simulink model "CAVE_MachE_speedCtrl"  (R2021b)
settings: configuration reference "ConfigSetDesktopFixedStep" (kept outside this file)
PreLoadFcn:
  | VSS_BICYCLE=Simulink.Variant('Dual=0');
  | VSS_DUAL=Simulink.Variant('Dual=1');
  | Dual=1;
  | load('DriveCycle2.mat')
PostLoadFcn:
  | if any(exist('dsrtsu_mdlpostloadfcn', 'file') ~= 0), dsrtsu_mdlpostloadfcn('Execute', bdroot); end
InitFcn:
  | , if any(exist('rtifpga_mdlclblib', 'file') ~= 0), rtifpga_mdlclblib('Init', bdroot); end,
  | , if any(exist('dsmpb_private', 'file') ~= 0), dsmpb_private('dsmpb_mdlclblib', 'Init', bdroot); end,
  | load('DriveCycle2.mat')
model workspace (MAT data in the model file):
  Gas = 0.383333333333
undefined symbols (not defined in the file or in its folder): AccelCmd, ActTqLF_Nm_, ActTqLR_Nm_, ActTqRF_Nm_, ActTqRR_Nm_, BattChargeLimitMaxPwr, BattChargeLimitSocBpts, BattChargeLimitTbl, BattChrgCapcty, BattDischargeLimitSocBpts, BattDischargeLimitTbl, BattDischargeMaxPwr, BattNumCellsParallel, BattNumCellsSeries, BattOpenVoltCapBpts, BattOpenVoltTbl, BattResistSocBpts, BattResistTbl, BattResistTempBpts, blkCmb_vertType_c1, BrakeMaxPrs, BrakeMaxTrq, ChassisDistCg2FrontAxle, ChassisDistCg2RearAxle, ChassisVehMass, CltchCmd, CoastDown, DecelCmd, DiffRatio, DiscIntNeverNeededParam, EnvGravCnst, EnvPrs, EnvTemp, FuelSpecificGrav, GearCmd, h, InitStates, lgSw, limitedMCT, MCT, MtrEffSpdBpts, MtrEffTbl, MtrEffTrqBpts, MtrPwrMax, MtrTrqMax, pMCT, Ref_speed, Ref_time, SteeringCmd, SupvsryCtrlRegenBrkCutOffTbl, SupvsryCtrlRegenSpdBpts, TestScnrioCycleNum, US06, vdynblks, VEH, vehdyntireFiala
libraries: VSIGenLib x65, simulink x54, etargetslib x38, dsmpblib x24, vehdynlibtire x12, autolibshared x9, vehdynlibsuspension x7, vehdynlibtirecommon x7, autolibutils x5, CarMaker4SL x4, VsrLibWheel x4, autolibpowerinfoutils x3
(part 5 of 14)

== system CAVE_MachE_speedCtrl/Vehicle Under Test/Vehicle/Vehicle Dynamics/Vehicle 14DOF/Brake Pressure ==
  BrkReq : Inport
  Bus Creator1 : BusCreator  Inputs=2
  Gain : Gain  Gain=BrakeMaxPrs
  Gain{1..4} (4 alike) : Gain  Gain=0.5
  Saturation{,1..3} (4 alike) : Saturate  UpperLimit=BrakeMaxPrs  LowerLimit=0  ZeroCross=off
  Signal Specification : SignalSpecification  Unit=Pa
  Terminator : Terminator
  Vector Concatenate2 : Concatenate  NumInputs=4
  BrakePrs : Outport  Unit=Pa
  wires:
  BrkReq/1 -> Gain/1, Bus Creator1/1  "BrkReq"
  Gain/1 -> Signal Specification/1
  Signal Specification/1 -> Gain2/1, Gain1/1, Bus Creator1/2  "BrkPrs"
  Bus Creator1/1 -> Terminator/1  "WhlBrk"
  Gain1/1 -> Gain4/1
  Gain2/1 -> Gain3/1
  Gain3/1 -> Saturation/1, Saturation1/1
  Gain4/1 -> Saturation2/1, Saturation3/1
  Vector Concatenate2/1 -> BrakePrs/1
  Saturation/1 -> Vector Concatenate2/1
  Saturation1/1 -> Vector Concatenate2/2
  Saturation2/1 -> Vector Concatenate2/3
  Saturation3/1 -> Vector Concatenate2/4

== system CAVE_MachE_speedCtrl/Vehicle Under Test/Vehicle/Vehicle Dynamics/Vehicle 14DOF/Steering ==
  SteeringCmd : Inport
  Constant : Constant  Value=0
  Kinematic Steering : vehdynlibsteering/Kinematic Steering  StrgType=Parallel  StrgRatioType=Constant  Loc=Front  NrmlFctr=1  TrckWdth=1.9  WhlBase=ChassisDistCg2FrontAxle+ChassisDistCg2RearAxle  Db=0  StrgRng=2.91*pi  StrgAngBpts="[-6.2832   -5.0265   -3.7699   -2.5133   -1.2566         0    1.2566    2.5133    3.7699    5.0265    6.2832]"  StrgRatioTbl=|  StrgRatio=16.8  StrgArmLngth=0.1  RckCsLngth=0.5  TieRodLngth=0.248  D=0.2  PnnRadius=0.0057  PnnRadiusTbl="[0.0055    0.0055    0.0056    0.0057    0.0058    0.0057    0.0057    0.0057    0.0056    0.0055    0.0055]"  RodLngth=0.1  ParaArmLngth=0.9  aMode=2
      | [13.5000   13.3750   13.2500   13.1250   13.0000   13.0000   13.0000   13.1250   13.2500   13.3750   13.5000
      | ]
  Terminator1 : Terminator
  Vector Concatenate : Concatenate
  Vector Concatenate1 : Concatenate
  Vector Concatenate2 : Concatenate
  WhlAng : Outport  Unit=rad
  wires:
  Kinematic Steering/1 -> Terminator1/1
  Vector Concatenate2/1 -> WhlAng/1
  Kinematic Steering/2 -> Vector Concatenate/1
  Vector Concatenate1/1 -> Vector Concatenate2/2  "RearWheelAngles"
  Vector Concatenate/1 -> Vector Concatenate2/1  "FrontWheelAngles"
  Constant/1 -> Vector Concatenate1/2, Vector Concatenate1/1
  Kinematic Steering/3 -> Vector Concatenate/2
  SteeringCmd/1 -> Kinematic Steering/1

== system CAVE_MachE_speedCtrl/Vehicle Under Test/Vehicle/Vehicle Dynamics/Vehicle 14DOF/Subsystem4 ==
  Cgxyzdot : Inport
  CgXYZ : Inport  Port=2
  CgXYZdot : Inport  Port=3
  angles : Inport  Port=4
  pqr : Inport  Port=5
  Cgaxyz : Inport  Port=6
  Beta : Inport  Port=7
  GeomXYZ : Inport  Port=8
  GeomXYZdot : Inport  Port=9
  Omega : Inport  Port=10
  Kappa : Inport  Port=11
  Alpha : Inport  Port=12
  XWheel : Inport  Port=13
  YWheel : Inport  Port=14
  dzWheel : Inport  Port=15
  Bus Creator : BusCreator  Inputs=26
  Bus Creator3 : BusCreator  Inputs=6
  Demux{,1..7} (8 alike) : Demux  Outputs=3
  Subsystem : Subsystem
  Chassis : Outport  VectorParamsAs1DForOutWhenUnconnected=off
  Wheels : Outport  Port=2  VectorParamsAs1DForOutWhenUnconnected=off
  wires:
  Bus Creator/1 -> Chassis/1  "Chassis"
  Omega/1 -> Bus Creator3/3  "Omega"
  dzWheel/1 -> Bus Creator3/6  "dZWheel"
  Kappa/1 -> Bus Creator3/1  "Kappa"
  Bus Creator3/1 -> Wheels/1  "Wheels"
  YWheel/1 -> Bus Creator3/5  "YWheel"
  XWheel/1 -> Bus Creator3/4  "XWheel"
  Alpha/1 -> Bus Creator3/2  "Alpha"
  Cgxyzdot/1 -> Subsystem/1(Cgxyzdot), Demux/1
  CgXYZ/1 -> Demux1/1
  CgXYZdot/1 -> Demux2/1
  angles/1 -> Subsystem/2(angles), Demux3/1
  pqr/1 -> Demux4/1
  Cgaxyz/1 -> Demux5/1
  GeomXYZdot/1 -> Demux7/1
  GeomXYZ/1 -> Demux6/1
  Demux/1 -> Bus Creator/1  "xdot"
  Demux/2 -> Bus Creator/2  "ydot"
  Demux/3 -> Bus Creator/3  "zdot"
  Demux1/1 -> Bus Creator/4  "X"
  Demux1/2 -> Bus Creator/5  "Y"
  Demux1/3 -> Bus Creator/6  "Z"
  Demux2/1 -> Bus Creator/7  "Xdot"
  Demux2/2 -> Bus Creator/8  "Ydot"
  Demux2/3 -> Bus Creator/9  "Zdot"
  Demux3/1 -> Bus Creator/10  "phi"
  Demux3/2 -> Bus Creator/11  "theta"
  Demux3/3 -> Bus Creator/12  "psi"
  Demux4/1 -> Bus Creator/13  "p"
  Demux4/2 -> Bus Creator/14  "q"
  Demux4/3 -> Bus Creator/15  "r"
  Demux5/1 -> Bus Creator/16  "ax"
  Demux5/2 -> Bus Creator/17  "ay"
  Demux5/3 -> Bus Creator/18  "az"
  Beta/1 -> Bus Creator/19  "Beta"
  Demux6/1 -> Bus Creator/20  "GeomX"
  Demux6/2 -> Bus Creator/21  "GeomY"
  Demux6/3 -> Bus Creator/22  "GeomZ"
  Demux7/1 -> Bus Creator/23  "GeomXdot"
  Demux7/2 -> Bus Creator/24  "GeomYdot"
  Demux7/3 -> Bus Creator/25  "GeomZdot"
  Subsystem/1(VehSpd) -> Bus Creator/26  "VehSpd"

== system CAVE_MachE_speedCtrl/Vehicle Under Test/Vehicle/Vehicle Dynamics/Vehicle 14DOF/Suspension ==
  Steering : Inport
  Vehicle : Inport  Port=2
  Wheel : Inport  Port=3
  Double Wishbone Suspension : Subsystem  VariantControl=1
      mask Display: image('suspdw.png');
  Independent Mapped Front Suspension Mapped Solid Axle Rear Suspension : Subsystem  VariantControl=2
      mask Display: image([imread('suspindmap.png');imread('suspsamap.png')]);
  MacPherson Front Suspension Solid Axle Rear Suspension : Subsystem  VariantControl=3
      mask Display: image([imread('suspmacp.png');imread('suspsacoil.png')]);
  MacPherson Suspension : Subsystem  VariantControl=4
      mask Display: image('suspmacp.png');
  Mapped Suspension : Subsystem  VariantControl=5
      mask Display: image('suspindmap.png');
  Suspension : Outport  VectorParamsAs1DForOutWhenUnconnected=off

== system CAVE_MachE_speedCtrl/Vehicle Under Test/Vehicle/Vehicle Dynamics/Vehicle 14DOF/Vehicle ==
  Suspension : Inport
  Wind : Inport  Port=2
  Variant Subsystem : Subsystem  Variant=on  VariantControlMode=label  LabelModeActiveChoice=1
  VehFdbk : Outport  VectorParamsAs1DForOutWhenUnconnected=off
  wires:
  Variant Subsystem/1(VehFdbk) -> VehFdbk/1  "VehFdbk"
  Wind/1 -> Variant Subsystem/2(Wind)
  Suspension/1 -> Variant Subsystem/1(Suspension)

== system CAVE_MachE_speedCtrl/Vehicle Under Test/Vehicle/Vehicle Dynamics/Vehicle 14DOF/Vehicle Routing ==
  Veh : Inport
  Bus Selector10 : BusSelector  OutputSignals=BdyFrm.Cg.Vel.xdot,BdyFrm.Cg.Vel.ydot,BdyFrm.Cg.Vel.zdot  OutputAsBus=on
  Bus Selector2 : BusSelector  OutputSignals=InertFrm.Cg.Disp.X,InertFrm.Cg.Disp.Y,InertFrm.Cg.Disp.Z  OutputAsBus=on
  Bus Selector3 : BusSelector  OutputSignals=InertFrm.Cg.Vel.Xdot,InertFrm.Cg.Vel.Ydot,InertFrm.Cg.Vel.Zdot  OutputAsBus=on
  Bus Selector4 : BusSelector  OutputSignals=BdyFrm.Cg.Acc.ax,BdyFrm.Cg.Acc.ay,BdyFrm.Cg.Acc.az  OutputAsBus=on
  Bus Selector5 : BusSelector  OutputSignals=InertFrm.Cg.Ang.phi,InertFrm.Cg.Ang.theta,InertFrm.Cg.Ang.psi  OutputAsBus=on
  Bus Selector6 : BusSelector  OutputSignals=BdyFrm.Cg.AngVel.p,BdyFrm.Cg.AngVel.q,BdyFrm.Cg.AngVel.r  OutputAsBus=on
  Bus Selector7 : BusSelector  OutputSignals=InertFrm.Geom.Disp.X,InertFrm.Geom.Disp.Y,InertFrm.Geom.Disp.Z  OutputAsBus=on
  Bus Selector8 : BusSelector  OutputSignals=InertFrm.Geom.Vel.Xdot,InertFrm.Geom.Vel.Ydot,InertFrm.Geom.Vel.Zdot  OutputAsBus=on
  Bus Selector9 : BusSelector  OutputSignals=BdyFrm.Geom.Ang.Beta
  Bus to Vector{1..8} (8 alike) : BusToVector
  Cgxyzdot : Outport  VectorParamsAs1DForOutWhenUnconnected=off
  CgXYZ : Outport  Port=2  VectorParamsAs1DForOutWhenUnconnected=off
  CgXYZdot : Outport  Port=3  VectorParamsAs1DForOutWhenUnconnected=off
  angles : Outport  Port=4  VectorParamsAs1DForOutWhenUnconnected=off
  pqr : Outport  Port=5  VectorParamsAs1DForOutWhenUnconnected=off
  Cgaxyz : Outport  Port=6  VectorParamsAs1DForOutWhenUnconnected=off
  Beta : Outport  Port=7  VectorParamsAs1DForOutWhenUnconnected=off
  GeomXYZ : Outport  Port=8  VectorParamsAs1DForOutWhenUnconnected=off
  GeomXYZdot : Outport  Port=9  VectorParamsAs1DForOutWhenUnconnected=off
  wires:
  Bus Selector3/1 -> Bus to Vector2/1
  Bus to Vector1/1 -> CgXYZ/1
  Bus to Vector5/1 -> pqr/1
  Bus Selector5/1 -> Bus to Vector4/1
  Bus Selector6/1 -> Bus to Vector5/1
  Bus to Vector4/1 -> angles/1
  Bus to Vector8/1 -> Cgxyzdot/1
  Bus Selector2/1 -> Bus to Vector1/1
  Bus Selector8/1 -> Bus to Vector7/1
  Bus to Vector6/1 -> GeomXYZ/1
  Bus Selector9/1 -> Beta/1  "<Beta>"
  Bus Selector4/1 -> Bus to Vector3/1
  Bus Selector10/1 -> Bus to Vector8/1
  Bus to Vector7/1 -> GeomXYZdot/1
  Bus to Vector3/1 -> Cgaxyz/1
  Bus Selector7/1 -> Bus to Vector6/1
  Bus to Vector2/1 -> CgXYZdot/1
  Veh/1 -> Bus Selector8/1, Bus Selector7/1, Bus Selector9/1, Bus Selector4/1, Bus Selector6/1, Bus Selector5/1, Bus Selector3/1, Bus Selector2/1, Bus Selector10/1

== system CAVE_MachE_speedCtrl/Vehicle Under Test/Vehicle/Vehicle Dynamics/Vehicle 14DOF/Wheel Routing ==
  Info : Inport
  Wheel : Inport  Port=2
  Bus Selector : BusSelector  OutputSignals=InertFrm.FrntAxl.Lft.Disp.Y,InertFrm.FrntAxl.Rght.Disp.Y,InertFrm.RearAxl.Lft.Disp.Y,InertFrm.RearAxl.Rght.Disp.Y
  Bus Selector1 : BusSelector  OutputSignals=InertFrm.FrntAxl.Lft.Disp.X,InertFrm.FrntAxl.Rght.Disp.X,InertFrm.RearAxl.Lft.Disp.X,InertFrm.RearAxl.Rght.Disp.X
  Bus Selector2 : BusSelector  OutputSignals=TireFrame.z,TireFrame.Omega,TireFrame.Kappa,TireFrame.Alpha
  Bus Selector3 : BusSelector  OutputSignals=InertFrm.FrntAxl.Lft.Disp.Z,InertFrm.FrntAxl.Rght.Disp.Z,InertFrm.RearAxl.Lft.Disp.Z,InertFrm.RearAxl.Rght.Disp.Z
  Bus Selector4 : BusSelector  OutputSignals=BdyFrm.FrntAxl.Lft.Disp.z,BdyFrm.FrntAxl.Rght.Disp.z,BdyFrm.RearAxl.Lft.Disp.z,BdyFrm.RearAxl.Rght.Disp.z
  Subtract : Sum  Inputs=-+-
  Vector Concatenate{1..4} (4 alike) : Concatenate  NumInputs=4
  Omega : Outport  PortDimensions=4  VectorParamsAs1DForOutWhenUnconnected=off
  Kappa : Outport  Port=2  PortDimensions=4  VectorParamsAs1DForOutWhenUnconnected=off
  Alpha : Outport  Port=3  PortDimensions=4  VectorParamsAs1DForOutWhenUnconnected=off
  XWheel : Outport  Port=4  Unit=m  VectorParamsAs1DForOutWhenUnconnected=off
  YWheel : Outport  Port=5  Unit=m  VectorParamsAs1DForOutWhenUnconnected=off
  ZWheel : Outport  Port=6  PortDimensions=4  VectorParamsAs1DForOutWhenUnconnected=off
  wires:
  Bus Selector1/4 -> Vector Concatenate2/4  "<X>"
  Bus Selector/1 -> Vector Concatenate1/1  "<Y>"
  Bus Selector1/3 -> Vector Concatenate2/3  "<X>"
  Bus Selector/4 -> Vector Concatenate1/4  "<Y>"
  Bus Selector1/2 -> Vector Concatenate2/2  "<X>"
  Bus Selector/3 -> Vector Concatenate1/3  "<Y>"
  Bus Selector/2 -> Vector Concatenate1/2  "<Y>"
  Vector Concatenate1/1 -> YWheel/1
  Bus Selector1/1 -> Vector Concatenate2/1  "<X>"
  Vector Concatenate2/1 -> XWheel/1
  Bus Selector2/1 -> Subtract/3  "<z>"
  Bus Selector2/2 -> Omega/1  "<Omega>"
  Bus Selector2/3 -> Kappa/1  "<Kappa>"
  Bus Selector2/4 -> Alpha/1  "<Alpha>"
  Wheel/1 -> Bus Selector2/1
  Subtract/1 -> ZWheel/1
  Info/1 -> Bus Selector1/1, Bus Selector4/1, Bus Selector3/1, Bus Selector/1
  Bus Selector3/2 -> Vector Concatenate3/2  "<Z>"
  Bus Selector3/3 -> Vector Concatenate3/3  "<Z>"
  Bus Selector3/4 -> Vector Concatenate3/4  "<Z>"
  Bus Selector3/1 -> Vector Concatenate3/1  "<Z>"
  Vector Concatenate3/1 -> Subtract/2
  Vector Concatenate4/1 -> Subtract/1
  Bus Selector4/1 -> Vector Concatenate4/1  "<z>"
  Bus Selector4/4 -> Vector Concatenate4/4  "<z>"
  Bus Selector4/3 -> Vector Concatenate4/3  "<z>"
  Bus Selector4/2 -> Vector Concatenate4/2  "<z>"

== system CAVE_MachE_speedCtrl/Vehicle Under Test/Vehicle/Vehicle Dynamics/Vehicle 14DOF/Wheels and Tires ==
  Suspension : Inport
  Axle Torque : Inport  Port=2
  Brake Press : Inport  Port=3  Unit=Pa
  Ground Input : Inport  Port=4
  Friction : Inport  Port=5  PortDimensions=4
  Bus Selector1 : BusSelector  OutputSignals=Whl.Ang,Whl.F,Whl.AngVel,Whl.xdot,Whl.ydot
  Constant3 : Constant  Value=zeros(4,1)
  Cont LPF : autolibutils/Cont LPF  wc=100*2*pi  aMode=2
      settings: SourceProductBaseCode=PW,DR,MT,UV,VE
  Cont LPF1 : autolibutils/Cont LPF  wc=100*2*pi  aMode=2
      settings: SourceProductBaseCode=PW,DR,MT,UV,VE
  Manual Switch6 : ManualSwitch
  Matrix Concatenate : Concatenate  NumInputs=3  Mode=Multidimensional array
  Reshape1 : Reshape
  Reshape2 : Reshape
  Saturation : Saturate  UpperLimit=10*9.81*2040  LowerLimit=-10*9.81*2040  ZeroCross=off
  Selector : Selector  NumberOfDimensions=2  InputPortWidth=3  IndexOptions=Index vector (dialog),Select all  Indices=[3],1  OutputSizes=1,1
  Selector1 : Selector  NumberOfDimensions=2  InputPortWidth=1  IndexOptions=Index vector (dialog),Select all  Indices=[3],1  OutputSizes=1,1
  Selector2 : Selector  NumberOfDimensions=2  InputPortWidth=3  IndexOptions=Index vector (dialog),Select all  Indices=3,1  OutputSizes=1,1
  Selector3 : Selector  NumberOfDimensions=2  InputPortWidth=3  IndexOptions=Index vector (dialog),Select all  Indices=1,1  OutputSizes=1,1
  Terminator{,1,3..5} (5 alike) : Terminator
  VDBS : Subsystem  VariantControl=0
  Wheels : Outport  VectorParamsAs1DForOutWhenUnconnected=off
  wires:
  VDBS/1(Wheels) -> Wheels/1  "Wheels"
  Bus Selector1/2 -> Selector/1  "<F>"
  VDBS/2(FrntAxlF) -> Terminator/1
  VDBS/3(RearAxlF) -> Terminator1/1
  VDBS/4(Omega) -> Terminator3/1
  VDBS/5(Mz) -> Terminator4/1
  Selector1/1 -> Reshape1/1
  Matrix Concatenate/1 -> VDBS/7(VehVel)
  Axle Torque/1 -> VDBS/3(AxleTrq)
  Selector2/1 -> VDBS/1(WheelAng)  "Wheel Angles"
  Constant3/1 -> Manual Switch6/1
  Manual Switch6/1 -> VDBS/2(CamberAng)  "Camber Angles"
  Selector/1 -> Reshape2/1
  Saturation/1 -> VDBS/5(Fz)
  Ground Input/1 -> VDBS/8(Ground Level)
  VDBS/7(SuspWhlVz) -> Matrix Concatenate/3  "zdot"
  Bus Selector1/1 -> Cont LPF1/1  "<Ang>"
  Selector3/1 -> Manual Switch6/2  "Camber Angles"
  Suspension/1 -> Bus Selector1/1
  Bus Selector1/4 -> Matrix Concatenate/1  "<xdot>"
  Bus Selector1/5 -> Matrix Concatenate/2  "<ydot>"
  VDBS/6(SuspWhlPz) -> Terminator5/1  "z"
  Reshape2/1 -> Cont LPF/1
  Bus Selector1/3 -> Selector1/1  "<AngVel>"
  Reshape1/1 -> VDBS/6(r)
  Brake Press/1 -> VDBS/4(BrkPrs)
  Friction/1 -> VDBS/9(Friction)
  Cont LPF/1 -> Saturation/1
  Cont LPF1/1 -> Selector3/1, Selector2/1

== system CAVE_MachE_speedCtrl/Vehicle Under Test/Vehicle/Vehicle Dynamics/Vehicle 7DOF/Brake Pressure ==
  BrkReq : Inport
  Bus Creator1 : BusCreator  Inputs=2
  Gain : Gain  Gain=BrakeMaxPrs
  Gain{1..4} (4 alike) : Gain  Gain=0.5
  Saturation{,1..3} (4 alike) : Saturate  UpperLimit=BrakeMaxPrs  LowerLimit=0  ZeroCross=off
  Signal Specification : SignalSpecification  Unit=Pa
  Terminator : Terminator
  Vector Concatenate2 : Concatenate  NumInputs=4
  BrakePrs : Outport  Unit=Pa
  wires:
  BrkReq/1 -> Gain/1, Bus Creator1/1  "BrkReq"
  Gain/1 -> Signal Specification/1
  Signal Specification/1 -> Gain2/1, Gain1/1, Bus Creator1/2  "BrkPrs"
  Bus Creator1/1 -> Terminator/1  "WhlBrk"
  Gain1/1 -> Gain4/1
  Gain2/1 -> Gain3/1
  Gain3/1 -> Saturation/1, Saturation1/1
  Gain4/1 -> Saturation2/1, Saturation3/1
  Vector Concatenate2/1 -> BrakePrs/1
  Saturation/1 -> Vector Concatenate2/1
  Saturation1/1 -> Vector Concatenate2/2
  Saturation2/1 -> Vector Concatenate2/3
  Saturation3/1 -> Vector Concatenate2/4

== system CAVE_MachE_speedCtrl/Vehicle Under Test/Vehicle/Vehicle Dynamics/Vehicle 7DOF/Longitudinal Wheels 4DOF ==
  WhlAng : Inport
  AxlTrq : Inport  Port=2
  BrkPrs : Inport  Port=3
  Gnd : Inport  Port=4  PortDimensions=4
  lam_mu : Inport  Port=5  PortDimensions=4
  VehFdbk : Inport  Port=6
  Axle Forces : Subsystem  Variant=on  VariantControlMode=label  LabelModeActiveChoice=1
  Bus Selector5 : BusSelector  OutputSignals=BdyFrm.Cg.AngVel.r
  Constant : vehdynlibtirecommon/Constant  const=220000  numWheels=4
      settings: SourceProductBaseCode=VE
  Constant3 : vehdynlibtirecommon/Constant  const=0  numWheels=4
      settings: SourceProductBaseCode=VE
  Terminator2 : Terminator
  Tire2Veh : Subsystem
  Tires : Subsystem
  Veh2Tire : Subsystem
  Velocity and Vertical Load : Subsystem  Variant=on  VariantControlMode=label  LabelModeActiveChoice=1
  Wheel Angles : Subsystem
  FrntAxlF : Outport  Unit=N  VectorParamsAs1DForOutWhenUnconnected=off
  RearAxlF : Outport  Port=2  Unit=N  VectorParamsAs1DForOutWhenUnconnected=off
  Omega : Outport  Port=3  VectorParamsAs1DForOutWhenUnconnected=off
  Kappa : Outport  Port=4  VectorParamsAs1DForOutWhenUnconnected=off
  Alpha : Outport  Port=5  VectorParamsAs1DForOutWhenUnconnected=off
  zAxle : Outport  Port=6  VectorParamsAs1DForOutWhenUnconnected=off
  wires:
  Wheel Angles/1(WhlAngB) -> Veh2Tire/5(WhlAng)
  Tires/1(Wheel) -> Tire2Veh/1(Wheel)
  lam_mu/1 -> Tires/9(lam_mu)
  Constant/1 -> Tires/7(TirePrs)
  Constant3/1 -> Wheel Angles/2(Camber), Tires/6(Camber)
  Veh2Tire/3(xdotAxle) -> Tires/3(Vx)  "Vx"
  Gnd/1 -> Tires/10(Gnd)
  VehFdbk/1 -> Bus Selector5/1, Velocity and Vertical Load/1(VehFdbk)
  AxlTrq/1 -> Veh2Tire/1(AxlTrq)
  Veh2Tire/1(T) -> Tires/1(AxlTrq)
  Veh2Tire/2(P) -> Tires/2(BrkPrs)
  BrkPrs/1 -> Veh2Tire/2(BrkPrs)
  Bus Selector5/1 -> Veh2Tire/3(r)  "<r>"
  Veh2Tire/6(zdotAxle) -> Terminator2/1
  WhlAng/1 -> Wheel Angles/1(WheelAng)  "FrontWheelAngles"
  Veh2Tire/4(ydotAxle) -> Tires/4(Vy)  "Vy"
  Veh2Tire/5(psidot) -> Tires/5(r)
  Velocity and Vertical Load/2(Fz) -> Tires/8(Fz)
  Velocity and Vertical Load/1(VehVel) -> Veh2Tire/4(VehVel)
  Axle Forces/1(FrntAxlF) -> FrntAxlF/1
  Axle Forces/2(RearAxlF) -> RearAxlF/1
  Tire2Veh/1(FwF) -> Axle Forces/1(F)
  Tire2Veh/2(FwR) -> Axle Forces/2(R)
  Tire2Veh/3(z) -> zAxle/1
  Tire2Veh/4(Omega) -> Omega/1
  Tire2Veh/5(Kappa) -> Kappa/1
  Tire2Veh/6(Alpha) -> Alpha/1

== system CAVE_MachE_speedCtrl/Vehicle Under Test/Vehicle/Vehicle Dynamics/Vehicle 7DOF/RototestDummy ==
  Bus Creator1 : BusCreator  Inputs=ActTqLF_Nm_,ActTqRF_Nm_,ActTqLR_Nm_,ActTqRR_Nm_
  Bus Creator2 : BusCreator  Inputs=Car Trq_T2WFL,Car Trq_T2WFR,Car Trq_T2WRL,Car Trq_T2WRR
  Bus Creator3 : BusCreator  Inputs=1
  Bus Creator4 : BusCreator  Inputs=1
  Bus Selector14 : BusSelector  OutputSignals=VehSpd
  Bus Selector15 : BusSelector  OutputSignals=TireFrame.Fx
  Constant{1..14} (14 alike) : Constant  Value=0
  Vector Concatenate3 : Concatenate  NumInputs=4
  CarTrqT2W : Outport
  AxleTrq : Outport  Port=2
  BrakePressed_flag : Outport  Port=3
  <VehSpd> : Outport  Port=4
  <Fx> : Outport  Port=5
  wires:
  Constant10/1 -> Bus Selector14/1  "VehSpd"
  Bus Creator4/1 -> Bus Creator3/1  "TireFrame"
  Bus Creator1/1 -> AxleTrq/1  "AxleTrq"
  Constant9/1 -> Bus Creator1/4  "ActTqRR_Nm_"
  Constant13/1 -> Bus Creator2/3  "CarTrq_T2WRL"
  Constant4/1 -> Vector Concatenate3/4
  Bus Creator3/1 -> Bus Selector15/1
  Vector Concatenate3/1 -> Bus Creator4/1  "Fx"
  Constant3/1 -> Vector Concatenate3/3
  Constant2/1 -> Vector Concatenate3/2
  Constant14/1 -> Bus Creator2/4  "CarTrq_T2WRR"
  Constant6/1 -> Bus Creator1/1  "ActTqLF_Nm_"
  Constant1/1 -> Vector Concatenate3/1
  Constant8/1 -> Bus Creator1/3  "ActTqLR_Nm_"
  Constant11/1 -> Bus Creator2/1  "CarTrq_T2WFL"
  Constant7/1 -> Bus Creator1/2  "ActTqRF_Nm_"
  Constant12/1 -> Bus Creator2/2  "CarTrq_T2WFR"
  Bus Creator2/1 -> CarTrqT2W/1  "CarTrqT2W"
  Bus Selector14/1 -> <VehSpd>/1  "<VehSpd>"
  Constant5/1 -> BrakePressed_flag/1  "BrakePressed_flag"
  Bus Selector15/1 -> <Fx>/1  "<Fx>"

== system CAVE_MachE_speedCtrl/Vehicle Under Test/Vehicle/Vehicle Dynamics/Vehicle 7DOF/Steering ==
  SteeringCmd : Inport
  Ground : Ground
  Kinematic Steering : vehdynlibsteering/Kinematic Steering  StrgType=Ackerman  StrgRatioType=Constant  Loc=Front  NrmlFctr=1  TrckWdth=1.9  WhlBase=ChassisDistCg2FrontAxle+ChassisDistCg2RearAxle  Db=0  StrgRng=3*pi  StrgAngBpts="[-6.2832   -5.0265   -3.7699   -2.5133   -1.2566         0    1.2566    2.5133    3.7699    5.0265    6.2832]"  StrgRatioTbl=|  StrgRatio=18  StrgArmLngth=0.1  RckCsLngth=0.5  TieRodLngth=0.248  D=0.2  PnnRadius=0.0057  PnnRadiusTbl="[0.0055    0.0055    0.0056    0.0057    0.0058    0.0057    0.0057    0.0057    0.0056    0.0055    0.0055]"  RodLngth=0.1  ParaArmLngth=0.9  aMode=2
      | [13.5000   13.3750   13.2500   13.1250   13.0000   13.0000   13.0000   13.1250   13.2500   13.3750   13.5000
      | ]
  Terminator1 : Terminator
  Vector Concatenate : Concatenate
  Vector Concatenate1 : Concatenate
  Vector Concatenate2 : Concatenate
  WhlAng : Outport  Unit=rad
  wires:
  Kinematic Steering/1 -> Terminator1/1
  Vector Concatenate2/1 -> WhlAng/1
  Kinematic Steering/2 -> Vector Concatenate/1
  Vector Concatenate1/1 -> Vector Concatenate2/2  "RearWheelAngles"
  Vector Concatenate/1 -> Vector Concatenate2/1  "FrontWheelAngles"
  Ground/1 -> Vector Concatenate1/2, Vector Concatenate1/1
  Kinematic Steering/3 -> Vector Concatenate/2
  SteeringCmd/1 -> Kinematic Steering/1

== system CAVE_MachE_speedCtrl/Vehicle Under Test/Vehicle/Vehicle Dynamics/Vehicle 7DOF/Subsystem4 ==
  Cgxyzdot : Inport
  CgXYZ : Inport  Port=2
  CgXYZdot : Inport  Port=3
  angles : Inport  Port=4
  pqr : Inport  Port=5
  Cgaxyz : Inport  Port=6
  Beta : Inport  Port=7
  GeomXYZ : Inport  Port=8
  GeomXYZdot : Inport  Port=9
  Omega : Inport  Port=10
  Kappa : Inport  Port=11
  Alpha : Inport  Port=12
  XWheel : Inport  Port=13
  YWheel : Inport  Port=14
  dzWheel : Inport  Port=15
  Bus Creator : BusCreator  Inputs=26
  Bus Creator3 : BusCreator  Inputs=6
  Demux{,1..7} (8 alike) : Demux  Outputs=3
  Subsystem : Subsystem
  Chassis : Outport  VectorParamsAs1DForOutWhenUnconnected=off
  Wheels : Outport  Port=2  VectorParamsAs1DForOutWhenUnconnected=off
  wires:
  Bus Creator/1 -> Chassis/1  "Chassis"
  Omega/1 -> Bus Creator3/3  "Omega"
  dzWheel/1 -> Bus Creator3/6  "dZWheel"
  Kappa/1 -> Bus Creator3/1  "Kappa"
  Bus Creator3/1 -> Wheels/1  "Wheels"
  YWheel/1 -> Bus Creator3/5  "YWheel"
  XWheel/1 -> Bus Creator3/4  "XWheel"
  Alpha/1 -> Bus Creator3/2  "Alpha"
  Cgxyzdot/1 -> Demux/1
  CgXYZ/1 -> Demux1/1
  CgXYZdot/1 -> Subsystem/1(CgXYZdot), Demux2/1
  angles/1 -> Subsystem/2(angles), Demux3/1
  pqr/1 -> Demux4/1
  Cgaxyz/1 -> Demux5/1
  GeomXYZdot/1 -> Demux7/1
  GeomXYZ/1 -> Demux6/1
  Demux/1 -> Bus Creator/1  "xdot"
  Demux/2 -> Bus Creator/2  "ydot"
  Demux/3 -> Bus Creator/3  "zdot"
  Demux1/1 -> Bus Creator/4  "X"
  Demux1/2 -> Bus Creator/5  "Y"
  Demux1/3 -> Bus Creator/6  "Z"
  Demux2/1 -> Bus Creator/7  "Xdot"
  Demux2/2 -> Bus Creator/8  "Ydot"
  Demux2/3 -> Bus Creator/9  "Zdot"
  Demux3/1 -> Bus Creator/10  "phi"
  Demux3/2 -> Bus Creator/11  "theta"
  Demux3/3 -> Bus Creator/12  "psi"
  Demux4/1 -> Bus Creator/13  "p"
  Demux4/2 -> Bus Creator/14  "q"
  Demux4/3 -> Bus Creator/15  "r"
  Demux5/1 -> Bus Creator/16  "ax"
  Demux5/2 -> Bus Creator/17  "ay"
  Demux5/3 -> Bus Creator/18  "az"
  Beta/1 -> Bus Creator/19  "Beta"
  Demux6/1 -> Bus Creator/20  "GeomX"
  Demux6/2 -> Bus Creator/21  "GeomY"
  Demux6/3 -> Bus Creator/22  "GeomZ"
  Demux7/1 -> Bus Creator/23  "GeomXdot"
  Demux7/2 -> Bus Creator/24  "GeomYdot"
  Demux7/3 -> Bus Creator/25  "GeomZdot"
  Subsystem/1(VehSpd) -> Bus Creator/26  "VehSpd"

== system CAVE_MachE_speedCtrl/Vehicle Under Test/Vehicle/Vehicle Dynamics/Vehicle 7DOF/Vehicle Body 3DOF External Longitudinal Wheels ==
  WhlAng : Inport
  "FwF " : Inport  Port=2
  "FwR " : Inport  Port=3
  WindXYZ : Inport  Port=4
  Friction : Inport  Port=5  Unit=1  PortDimensions=4
  Bicycle : Subsystem  VariantControl=0
  Dual : Subsystem  VariantControl=1
  " Info" : Outport  VectorParamsAs1DForOutWhenUnconnected=off
  " XWheel" : Outport  Port=2  VectorParamsAs1DForOutWhenUnconnected=off
  " YWheel" : Outport  Port=3  VectorParamsAs1DForOutWhenUnconnected=off

== system CAVE_MachE_speedCtrl/Vehicle Under Test/Vehicle/Vehicle Dynamics/Vehicle Longitudinal/Brake Pressure ==
  BrkReq : Inport
  Bus Creator1 : BusCreator  Inputs=2
  Gain : Gain  Gain=BrakeMaxPrs
  Gain{1..4} (4 alike) : Gain  Gain=0.5
  Saturation{,1..3} (4 alike) : Saturate  UpperLimit=BrakeMaxPrs  LowerLimit=0  ZeroCross=off
  Signal Specification : SignalSpecification  Unit=Pa
  Terminator : Terminator
  Vector Concatenate2 : Concatenate  NumInputs=4
  BrakePrs : Outport  Unit=Pa
  wires:
  BrkReq/1 -> Gain/1, Bus Creator1/1  "BrkReq"
  Gain/1 -> Signal Specification/1
  Signal Specification/1 -> Gain2/1, Gain1/1, Bus Creator1/2  "BrkPrs"
  Bus Creator1/1 -> Terminator/1  "WhlBrk"
  Gain1/1 -> Gain4/1
  Gain2/1 -> Gain3/1
  Gain3/1 -> Saturation/1, Saturation1/1
  Gain4/1 -> Saturation2/1, Saturation3/1
  Vector Concatenate2/1 -> BrakePrs/1
  Saturation/1 -> Vector Concatenate2/1
  Saturation1/1 -> Vector Concatenate2/2
  Saturation2/1 -> Vector Concatenate2/3
  Saturation3/1 -> Vector Concatenate2/4

== system CAVE_MachE_speedCtrl/Vehicle Under Test/Vehicle/Vehicle Dynamics/Vehicle Longitudinal/Longitudinal Wheels ==
  BrkPrs : Inport
  AxleTorq : Inport  Port=2
  Bus Creator : BusCreator  Inputs=3
  Bus Selector : BusSelector  OutputSignals=WhlRearInfo,Omega3,Omega4
  Bus Selector1 : BusSelector  OutputSignals=WhlFrontInfo,Omega1,Omega2
  Front Diff Wheels : Subsystem
  Rear Wheels : Subsystem
  Vector Concatenate : Concatenate  NumInputs=4
  FrontAxle : PMIOPort  Side=Right
  RearAxle : PMIOPort  Port=2  Side=Right
  Whl : Outport
  wires:
  Rear Wheels/1(Info) -> Bus Selector/1  "WhlRearInfo"
  Front Diff Wheels/1(Info) -> Bus Selector1/1  "WhlFrontInfo"
  Bus Creator/1 -> Whl/1  "Whl"
  BrkPrs/1 -> Front Diff Wheels/1(BrkPrs), Rear Wheels/1(BrkPrs)
  AxleTorq/1 -> Front Diff Wheels/2(AxleTorq)
  Bus Selector/2 -> Vector Concatenate/3  "<Omega3>"
  Bus Selector1/1 -> Bus Creator/1  "<WhlFrontInfo>"
  Bus Selector1/2 -> Vector Concatenate/1  "<Omega1>"
  Bus Selector1/3 -> Vector Concatenate/2  "<Omega2>"
  Bus Selector/3 -> Vector Concatenate/4  "<Omega4>"
  Bus Selector/1 -> Bus Creator/2  "<WhlRearInfo>"
  Vector Concatenate/1 -> Bus Creator/3  "Omega"
  connections:
  RearAxle/RConn1 -- Rear Wheels/RConn1
  Front Diff Wheels/RConn1 -- FrontAxle/RConn1

== system CAVE_MachE_speedCtrl/Vehicle Under Test/Vehicle/Vehicle Dynamics/Vehicle Longitudinal/RototestDummy ==
  Bus Creator1 : BusCreator  Inputs=ActTqLF_Nm_,ActTqRF_Nm_,ActTqLR_Nm_,ActTqRR_Nm_
  Bus Creator2 : BusCreator  Inputs=Car Trq_T2WFL,Car Trq_T2WFR,Car Trq_T2WRL,Car Trq_T2WRR
  Bus Creator3 : BusCreator  Inputs=1
  Bus Creator4 : BusCreator  Inputs=1
  Bus Selector14 : BusSelector  OutputSignals=VehSpd
  Bus Selector15 : BusSelector  OutputSignals=TireFrame.Fx
  Constant{1..14} (14 alike) : Constant  Value=0
  Vector Concatenate3 : Concatenate  NumInputs=4
  CarTrqT2W : Outport
  AxleTrq : Outport  Port=2
  BrakePressed_flag : Outport  Port=3
  <VehSpd> : Outport  Port=4
  <Fx> : Outport  Port=5
  wires:
  Constant10/1 -> Bus Selector14/1  "VehSpd"
  Bus Creator4/1 -> Bus Creator3/1  "TireFrame"
  Bus Creator1/1 -> AxleTrq/1  "AxleTrq"
  Constant9/1 -> Bus Creator1/4  "ActTqRR_Nm_"
  Constant13/1 -> Bus Creator2/3  "CarTrq_T2WRL"
  Constant4/1 -> Vector Concatenate3/4
  Bus Creator3/1 -> Bus Selector15/1
  Vector Concatenate3/1 -> Bus Creator4/1  "Fx"
  Constant3/1 -> Vector Concatenate3/3
  Constant2/1 -> Vector Concatenate3/2
  Constant14/1 -> Bus Creator2/4  "CarTrq_T2WRR"
  Constant6/1 -> Bus Creator1/1  "ActTqLF_Nm_"
  Constant1/1 -> Vector Concatenate3/1
  Constant8/1 -> Bus Creator1/3  "ActTqLR_Nm_"
  Constant11/1 -> Bus Creator2/1  "CarTrq_T2WFL"
  Constant7/1 -> Bus Creator1/2  "ActTqRF_Nm_"
  Constant12/1 -> Bus Creator2/2  "CarTrq_T2WFR"
  Bus Creator2/1 -> CarTrqT2W/1  "CarTrqT2W"
  Bus Selector14/1 -> <VehSpd>/1  "<VehSpd>"
  Constant5/1 -> BrakePressed_flag/1  "BrakePressed_flag"
  Bus Selector15/1 -> <Fx>/1  "<Fx>"

== system CAVE_MachE_speedCtrl/Vehicle Under Test/Vehicle/Vehicle Dynamics/Vehicle Longitudinal/Vehicle Body ==
  RoadGrade : Inport
  WindX : Inport  Port=2
  Logitudinal Vehicle Body : Subsystem
  Subsystem1 : Subsystem
      mask Display: disp('')
  FrontAxle : PMIOPort  Side=Left
  RearDiff : PMIOPort  Port=2  Side=Left
  Chassis : Outport
  wires:
  Logitudinal Vehicle Body/1(VehSpd) -> Subsystem1/1(VehSpd)
  Logitudinal Vehicle Body/2(VehDist) -> Subsystem1/2(VehDist)
  Logitudinal Vehicle Body/3(FrontAxleFrc) -> Subsystem1/3(FrontAxleFrc)
  Logitudinal Vehicle Body/4(RearAxleFrc) -> Subsystem1/4(RearAxleFrc)
  Subsystem1/1(ChassisPlant) -> Chassis/1
  RoadGrade/1 -> Logitudinal Vehicle Body/1(RoadGrade)
  WindX/1 -> Logitudinal Vehicle Body/2(WindVel)
  connections:
  RearDiff/RConn1 -- Logitudinal Vehicle Body/LConn2
  FrontAxle/RConn1 -- Logitudinal Vehicle Body/LConn1

== system CAVE_MachE_speedCtrl/Vehicle Under Test/Vehicle/Actuation and Outputs/MOOG Brake Actuator/ CAN Settings/ CAN diagnostic Counter ==
  RX Counter : Inport
  Compare To Constant3 : simulink/Logic and Bit Operations/Compare To Constant  relop=<=  const=TimeOutDuration  OutDataTypeStr=boolean
  Memory2 : Memory  InheritSampleTime=on
  Relational Operator2 : RelationalOperator  Operator=~=  OutDataTypeStr=boolean  RndMeth=Nearest
  Timer : Subsystem
  CommsOKFlag : Outport
  wires:
  Relational Operator2/1 -> Timer/1(Reset)
  Timer/1(Timer) -> Compare To Constant3/1
  RX Counter/1 -> Relational Operator2/1, Memory2/1
  Memory2/1 -> Relational Operator2/2
  Compare To Constant3/1 -> CommsOKFlag/1

== system CAVE_MachE_speedCtrl/Vehicle Under Test/Vehicle/Actuation and Outputs/MOOG Brake Actuator/MOOG Interface/Max Stop Adjustment ==
  In1 : Inport
  Enable : EnablePort
  MaxStopOffset : Constant  Value=-5500
  Sum3 : Sum  Inputs=|++
  Out1 : Outport  InitialOutput=[0]
  wires:
  MaxStopOffset/1 -> Sum3/2
  In1/1 -> Sum3/1
  Sum3/1 -> Out1/1

== system CAVE_MachE_speedCtrl/Vehicle Under Test/Vehicle/Actuation and Outputs/MOOG Brake Actuator/MOOG Interface/Min Stop Adjustment ==
  In1 : Inport
  Enable : EnablePort
  MinStopOffset : Constant  Value=3500
  Sum3 : Sum  Inputs=|++
  Out1 : Outport  InitialOutput=[0]
  wires:
  In1/1 -> Sum3/1
  Sum3/1 -> Out1/1
  MinStopOffset/1 -> Sum3/2

== system CAVE_MachE_speedCtrl/Vehicle Under Test/Vehicle/Actuation and Outputs/MOOG Brake Actuator/MOOG Interface/Rising edge ==
  In : Inport
  Memory : Memory  InheritSampleTime=on
  Sum3 : Sum  Inputs=|+-
  Out : Outport
  wires:
  In/1 -> Memory/1, Sum3/1
  Memory/1 -> Sum3/2
  Sum3/1 -> Out/1

== system CAVE_MachE_speedCtrl/Vehicle Under Test/Vehicle/Actuation and Outputs/MOOG Brake Actuator/MOOG Interface/Rising edge1 ==
  In : Inport
  Memory : Memory  InheritSampleTime=on
  Sum3 : Sum  Inputs=|+-
  Out : Outport
  wires:
  In/1 -> Memory/1, Sum3/1
  Memory/1 -> Sum3/2
  Sum3/1 -> Out/1

== system CAVE_MachE_speedCtrl/Vehicle Under Test/Vehicle/Battery/Battery/Lithium Ion Battery Pack1/Datasheet Battery Internal ==
  BattCurr : Inport
  BattTemp : Inport  Port=2
  Constant1 : Constant  Value=BattCapInit
  Datasheet Battery : Subsystem  AncestorBlock=autolibbatterycommon/Datasheet Battery
  LdCurrFeed : Outport  VectorParamsAs1DForOutWhenUnconnected=off
  OutVoltUnfilt : Outport  Port=2  VectorParamsAs1DForOutWhenUnconnected=off
  LdAmpHr : Outport  Port=3  VectorParamsAs1DForOutWhenUnconnected=off
  BattSoc : Outport  Port=4  VectorParamsAs1DForOutWhenUnconnected=off
  BattPwrLoss : Outport  Port=5  VectorParamsAs1DForOutWhenUnconnected=off
  wires:
  Datasheet Battery/5(BattPwrLoss) -> BattPwrLoss/1
  Datasheet Battery/1(LdCurrFeed) -> LdCurrFeed/1
  Datasheet Battery/2(OutVoltUnfilt) -> OutVoltUnfilt/1
  Datasheet Battery/3(LdAmpHr) -> LdAmpHr/1
  Datasheet Battery/4(BattSoc) -> BattSoc/1
  BattTemp/1 -> Datasheet Battery/3(BattTemp)
  BattCurr/1 -> Datasheet Battery/2(BattCurr)
  Constant1/1 -> Datasheet Battery/1(CapInit)

== system CAVE_MachE_speedCtrl/Vehicle Under Test/Vehicle/Driver and Drive Cycle/Driver and PI with FF Control/Speed controller set/In-house CAVE ==
  note: BrakeSwitch
  RefSpd [km/hr] : Inport
  In2 : Inport  Port=2
  In-house Speed Controller : Subsystem
  AccelPedalCmd : Outport
  BrakePedalCmd : Outport  Port=2
  Out3 : Outport  Port=3
  wires:
  In-house Speed Controller/3(BrakeSwitch) -> Out3/1
  In-house Speed Controller/2(BrakePedalPos) -> BrakePedalCmd/1  "BrakePedalCmd"
  RefSpd [km/hr]/1 -> In-house Speed Controller/1(RefSpd)
  In2/1 -> In-house Speed Controller/2(VehicleSpeed)
  In-house Speed Controller/1(AcceleratorPedalPos) -> AccelPedalCmd/1  "AccelPedalCmd"

== system CAVE_MachE_speedCtrl/Vehicle Under Test/Vehicle/Driver and Drive Cycle/Driver and PI with FF Control/Speed controller set/PIF ==
  RefSpd [km/hr] : Inport
  In2 : Inport  Port=2
  Compare To Constant1 : simulink/Logic and Bit Operations/Compare To Constant  relop=<=  const=0.1  OutDataTypeStr=boolean  ZeroCross=off
  Constant : Constant  Value=0
  Constant1 : Constant  Value=0
  Gain : Gain  Gain=1/3.6
  Gain1 : Gain  Gain=1/3.6
  Gain2 : Gain  Gain=100
  Gain3 : Gain  Gain=100
  Longitudinal Driver : autolibshared/Longitudinal Driver  cntrlType=PI  shftType=None  velUnits=m/s  gearOut=off  Kp=2.5  Ki=1  Kff=.1*0.35  Kg=0  VehVelVec=[0 100]  KffVec=[.1 .1]  KpVec=[10 10]  KiVec=[5 5]  KgVec=[0 0]  m=1500  Kpt=3000  tau=.1  L=2  aR=200  bR=2.5  cR=.5  g=9.81  vnom=1  Kaw=1  tauerr=.01  tauPt=2  GearInit=0  tShift=.1  pdlVec=[0.1 0.4 0.5 0.9]  upShftTbl=[-1 12.9375 26.4375 39.9375 51.18749999999999 62.4375 72.84375 83.25;-1 16.3125 29.8125 43.3125 54.5624 65.8125 76.78125 87.75;-1 19.6875 33.1875 46.68749999999999 57.9375 69.1875 80.71875 92.25;-1 33 52.5 77.25 100.5 138.75 161.875 185]  dwnShftTbl=[1 9.5625 23.0625 36.5625 47.8125 59.0625 68.90625 78.75;1 12.9375 26.4375 39.9375 51.18749999999999 62.4375 72.84375 83.25;1 16.3125 29.8125 43.3125 54.562499 65.8125 76.78125 87.75;1 19.6875 33.1875 46.68749999999999 57.9375 69.1875 80.71875 92.25]  tClutch=.5  tRev=.5  tPark=120  aMode=2  UpGearVec="[0  1  2  3  4  5  6  7]"  DownGearVec="[1  2  3  4  5  6  7  8]"
      settings: SourceProductBaseCode=PW,DR,MT,UV,VE
  Lowpass Filter : TransferFcn  Denominator=[.01 1]
  Min threshold for Brake switch : Constant  Value=0
  Relational Operator : RelationalOperator  Operator=>  OutDataTypeStr=boolean  RndMeth=Nearest
  Switch3 : Switch  Criteria=u2 > Threshold
  Switch4 : Switch  Criteria=u2 > Threshold
  Terminator : Terminator
  standstill brake [0,1] : Constant  Value=0.5
  AccelPedalCmd : Outport
  BrakePedalCmd : Outport  Port=2
  Out3 : Outport  Port=3
  wires:
  Gain1/1 -> Longitudinal Driver/2
  Min threshold for Brake switch/1 -> Relational Operator/2
  Relational Operator/1 -> Out3/1  "BrakeSwitch"
  Longitudinal Driver/3 -> Switch4/3, Relational Operator/1  "BrakePedalPosPre_pct"
  Gain/1 -> Compare To Constant1/1, Longitudinal Driver/1
  Constant1/1 -> Longitudinal Driver/3
  RefSpd [km/hr]/1 -> Gain/1
  In2/1 -> Lowpass Filter/1
  Gain3/1 -> BrakePedalCmd/1  "BrakePedalCmd"
  Gain2/1 -> AccelPedalCmd/1  "AccelPedalCmd"
  Longitudinal Driver/1 -> Terminator/1
  Longitudinal Driver/2 -> Switch3/3  "AcceleratorPedalPosPre_pct"
  Constant/1 -> Switch3/1
  Compare To Constant1/1 -> Switch4/2, Switch3/2
  standstill brake [0,1]/1 -> Switch4/1
  Switch3/1 -> Gain2/1  "AcceleratorPedalPos_pct"
  Switch4/1 -> Gain3/1  "BrakePedalPos_pct"
  Lowpass Filter/1 -> Gain1/1  "VS_Flt"

== system CAVE_MachE_speedCtrl/Vehicle Under Test/Vehicle/Driver and Drive Cycle/Driver and PI with FF Control/Speed controller set/Predictive ==
  RefSpd [km/hr] : Inport
  In2 : Inport  Port=2
  Compare To Constant1 : simulink/Logic and Bit Operations/Compare To Constant  relop=<=  const=0.1  OutDataTypeStr=boolean  ZeroCross=off
  Constant : Constant  Value=0
  Constant1 : Constant  Value=0
  Gain : Gain  Gain=1/3.6
  Gain1 : Gain  Gain=1/3.6
  Gain4 : Gain  Gain=100
  Gain5 : Gain  Gain=100
  Longitudinal Driver : autolibshared/Longitudinal Driver  cntrlType=Predictive  shftType=None  velUnits=m/s  gearOut=off  Kp=10  Ki=5  Kff=.1  Kg=0  VehVelVec=[0 100]  KffVec=[.1 .1]  KpVec=[10 10]  KiVec=[5 5]  KgVec=[0 0]  m=2040  Kpt=6500  tau=0.1  L=3  aR=200/10  bR=2.5/100  cR=.3  g=9.807  vnom=5  Kaw=1  tauerr=.01  tauPt=2  GearInit=0  tShift=.1  pdlVec=[0.1 0.4 0.5 0.9]  upShftTbl=[-1 12.9375 26.4375 39.9375 51.18749999999999 62.4375 72.84375 83.25;-1 16.3125 29.8125 43.3125 54.5624 65.8125 76.78125 87.75;-1 19.6875 33.1875 46.68749999999999 57.9375 69.1875 80.71875 92.25;-1 33 52.5 77.25 100.5 138.75 161.875 185]  dwnShftTbl=[1 9.5625 23.0625 36.5625 47.8125 59.0625 68.90625 78.75;1 12.9375 26.4375 39.9375 51.18749999999999 62.4375 72.84375 83.25;1 16.3125 29.8125 43.3125 54.562499 65.8125 76.78125 87.75;1 19.6875 33.1875 46.68749999999999 57.9375 69.1875 80.71875 92.25]  tClutch=.5  tRev=.5  tPark=120  aMode=2  UpGearVec="[0  1  2  3  4  5  6  7]"  DownGearVec="[1  2  3  4  5  6  7  8]"
      settings: SourceProductBaseCode=PW,DR,MT,UV,VE
  Lowpass Filter : TransferFcn  Denominator=[.02 1]
  Min threshold for Brake switch : Constant  Value=0
  Relational Operator : RelationalOperator  Operator=>  OutDataTypeStr=boolean  RndMeth=Nearest
  Switch3 : Switch  Criteria=u2 > Threshold
  Switch4 : Switch  Criteria=u2 > Threshold
  Terminator : Terminator
  standstill brake [0,1] : Constant  Value=0.5
  AccelPedalCmd : Outport
  BrakePedalCmd : Outport  Port=2
  Out3 : Outport  Port=3
  wires:
  Gain1/1 -> Longitudinal Driver/2
  Min threshold for Brake switch/1 -> Relational Operator/2
  Relational Operator/1 -> Out3/1  "BrakeSwitch"
  Constant1/1 -> Longitudinal Driver/3
  RefSpd [km/hr]/1 -> Gain/1
  In2/1 -> Lowpass Filter/1
  Longitudinal Driver/1 -> Terminator/1
  standstill brake [0,1]/1 -> Switch4/1
  Longitudinal Driver/3 -> Switch4/3, Relational Operator/1  "BrakePedalPosPre_pct"
  Switch4/1 -> Gain5/1  "BrakePedalPos_pct"
  Switch3/1 -> Gain4/1  "AcceleratorPedalPos_pct"
  Compare To Constant1/1 -> Switch4/2, Switch3/2
  Constant/1 -> Switch3/1
  Gain4/1 -> AccelPedalCmd/1  "AccelPedalCmd"
  Gain/1 -> Compare To Constant1/1, Longitudinal Driver/1
  Gain5/1 -> BrakePedalCmd/1  "BrakePedalCmd"
  Longitudinal Driver/2 -> Switch3/3  "AcceleratorPedalPosPre_pct"
  Lowpass Filter/1 -> Gain1/1  "VS_Flt"

== system CAVE_MachE_speedCtrl/Vehicle Under Test/Vehicle/Driver and Drive Cycle/Driver and PI with FF Control/Speed controller set/Speed tracking controller ==
  RefSpd [km/hr] : Inport
  In2 : Inport  Port=2
  In-house CAVE : Subsystem  VariantControl=varaint1
  PIF : Subsystem  VariantControl=varaint2
  Predictive : Subsystem  VariantControl=varaint3
  AccelPedalCmd : Outport
  BrakePedalCmd : Outport  Port=2
  Out3 : Outport  Port=3

== system CAVE_MachE_speedCtrl/Vehicle Under Test/Vehicle/Powertrain Supervisory Controller /Engine Torque Command/Accel Pedal to Traction Wheel Torque Request1/Max Motor Torque ==
  MtrSpd : Inport
  Constant : Constant  Value=MtrPwrMax
  Divide : Product  Inputs=*/
  Saturation : Saturate  UpperLimit=MtrTrqMax  LowerLimit=0
  Saturation1 : Saturate  UpperLimit=inf  LowerLimit=1
  MtrTrqMax : Outport
  wires:
  Saturation/1 -> MtrTrqMax/1
  Saturation1/1 -> Divide/2
  Divide/1 -> Saturation/1
  MtrSpd/1 -> Saturation1/1
  Constant/1 -> Divide/1

== system CAVE_MachE_speedCtrl/Vehicle Under Test/Vehicle/Powertrain Supervisory Controller /Engine Torque Command/Motor Torque Arbitration and Power Management/Power Management ==
  note: Power Management algorithm:
      | - Estimate Elec power based on mech power using efficiency map
      | - Check if Elec power is within battery power limits
      | - If power within limit , use motor torque command
      | - If power limit exceeded, use limited motor torque
      | - For low Mot Spd, MotPwrReq will be a small number.  Pass through torque command until Mot Spd > 2.
  BattPwrDischrgLmt : Inport
  BattPwrChrgLmt : Inport  Port=2
  MotSpd : Inport  Port=3
  MotTrqCmd : Inport  Port=4
  Abs : Abs
  Check Within Limits : Subsystem
  Compare To Constant : simulink/Logic and Bit Operations/Compare To Constant  relop=<  const=2  OutDataTypeStr=boolean
  ElecToMechPwr : Product  Inputs=*/
  Mech to Elec Power Estimate : Subsystem
  MechPwrToTrq : Product  Inputs=*/
  Switch : Switch  Criteria=u2 > Threshold
  Switch1 : Switch  Criteria=u2 > Threshold
  Torque Limit : Subsystem
  div0protect - poly : autolibutils/div0protect - poly  thresh=2  ZeroCross1=off  aMode=aMode
      settings: SourceProductBaseCode=PW,DR,MT,UV,VE
  MotTrqCmdFinal : Outport  VectorParamsAs1DForOutWhenUnconnected=off
  wires:
  Compare To Constant/1 -> Switch1/2
  Abs/1 -> Compare To Constant/1
  Switch1/1 -> Torque Limit/1(MotTrq)
  Check Within Limits/1(InLimit) -> Switch/2
  Switch/1 -> Switch1/3
  Check Within Limits/2(y) -> ElecToMechPwr/1
  BattPwrChrgLmt/1 -> Check Within Limits/3(lo)
  Mech to Elec Power Estimate/1(MotPwrElecReq) -> Check Within Limits/2(u)
  BattPwrDischrgLmt/1 -> Check Within Limits/1(up)
  Torque Limit/1(MotTrqCmd) -> MotTrqCmdFinal/1
  MechPwrToTrq/1 -> Switch/3
  ElecToMechPwr/1 -> MechPwrToTrq/1
  Mech to Elec Power Estimate/2(Eff2k) -> ElecToMechPwr/2
  div0protect - poly/1 -> MechPwrToTrq/2
  MotTrqCmd/1 -> Mech to Elec Power Estimate/1(MotTrqCmd), Switch1/1, Switch/1
  MotSpd/1 -> Abs/1, Mech to Elec Power Estimate/2(MotSpd), div0protect - poly/1, Torque Limit/2(MotSpd)

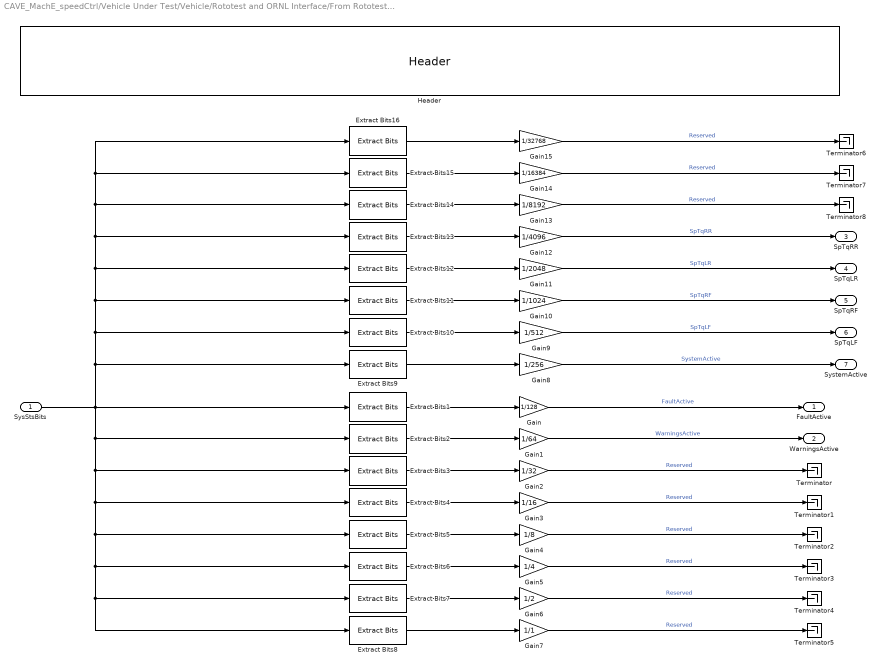
== system CAVE_MachE_speedCtrl/Vehicle Under Test/Vehicle/Rototest and ORNL Interface/From Rototest/RotoTestEthRX/Depacker ==
  SysStsBits : Inport
  Extract Bits1 : simulink/Logic and Bit Operations/Extract Bits  bitsToExtract=Range of bits  numBits=8  bitIdxRange=[7]  outScalingMode=Preserve fixed-point scaling
  Extract Bits10 : simulink/Logic and Bit Operations/Extract Bits  bitsToExtract=Range of bits  numBits=8  bitIdxRange=[9]  outScalingMode=Preserve fixed-point scaling
  Extract Bits11 : simulink/Logic and Bit Operations/Extract Bits  bitsToExtract=Range of bits  numBits=8  bitIdxRange=[10]  outScalingMode=Preserve fixed-point scaling
  Extract Bits12 : simulink/Logic and Bit Operations/Extract Bits  bitsToExtract=Range of bits  numBits=8  bitIdxRange=[11]  outScalingMode=Preserve fixed-point scaling
  Extract Bits13 : simulink/Logic and Bit Operations/Extract Bits  bitsToExtract=Range of bits  numBits=8  bitIdxRange=[12]  outScalingMode=Preserve fixed-point scaling
  Extract Bits14 : simulink/Logic and Bit Operations/Extract Bits  bitsToExtract=Range of bits  numBits=8  bitIdxRange=[13]  outScalingMode=Preserve fixed-point scaling
  Extract Bits15 : simulink/Logic and Bit Operations/Extract Bits  bitsToExtract=Range of bits  numBits=8  bitIdxRange=[14]  outScalingMode=Preserve fixed-point scaling
  Extract Bits16 : simulink/Logic and Bit Operations/Extract Bits  bitsToExtract=Range of bits  numBits=8  bitIdxRange=[15]  outScalingMode=Preserve fixed-point scaling
  Extract Bits2 : simulink/Logic and Bit Operations/Extract Bits  bitsToExtract=Range of bits  numBits=8  bitIdxRange=[6]  outScalingMode=Preserve fixed-point scaling
  Extract Bits3 : simulink/Logic and Bit Operations/Extract Bits  bitsToExtract=Range of bits  numBits=8  bitIdxRange=[5]  outScalingMode=Preserve fixed-point scaling
  Extract Bits4 : simulink/Logic and Bit Operations/Extract Bits  bitsToExtract=Range of bits  numBits=8  bitIdxRange=[4]  outScalingMode=Preserve fixed-point scaling
  Extract Bits5 : simulink/Logic and Bit Operations/Extract Bits  bitsToExtract=Range of bits  numBits=8  bitIdxRange=[3]  outScalingMode=Preserve fixed-point scaling
  Extract Bits6 : simulink/Logic and Bit Operations/Extract Bits  bitsToExtract=Range of bits  numBits=8  bitIdxRange=[2]  outScalingMode=Preserve fixed-point scaling
  Extract Bits7 : simulink/Logic and Bit Operations/Extract Bits  bitsToExtract=Range of bits  numBits=8  bitIdxRange=[1]  outScalingMode=Preserve fixed-point scaling
  Extract Bits8 : simulink/Logic and Bit Operations/Extract Bits  bitsToExtract=Range of bits  numBits=8  bitIdxRange=[0]  outScalingMode=Preserve fixed-point scaling
  Extract Bits9 : simulink/Logic and Bit Operations/Extract Bits  bitsToExtract=Range of bits  numBits=8  bitIdxRange=[8]  outScalingMode=Preserve fixed-point scaling
  Gain : Gain  Gain=1/128
  Gain1 : Gain  Gain=1/64
  Gain10 : Gain  Gain=1/1024
  Gain11 : Gain  Gain=1/2048
  Gain12 : Gain  Gain=1/4096
  Gain13 : Gain  Gain=1/8192
  Gain14 : Gain  Gain=1/16384
  Gain15 : Gain  Gain=1/32768
  Gain2 : Gain  Gain=1/32
  Gain3 : Gain  Gain=1/16
  Gain4 : Gain  Gain=1/8
  Gain5 : Gain  Gain=1/4
  Gain6 : Gain  Gain=1/2
  Gain7 : Gain  Gain=1/1
  Gain8 : Gain  Gain=1/256
  Gain9 : Gain  Gain=1/512
  Header : VSIGenLib/Header  not=''
  Terminator{,1..8} (9 alike) : Terminator
  FaultActive : Outport
  WarningsActive : Outport  Port=2
  SpTqRR : Outport  Port=3
  SpTqLR : Outport  Port=4
  SpTqRF : Outport  Port=5
  SpTqLF : Outport  Port=6
  SystemActive : Outport  Port=7
  wires:
  Gain5/1 -> Terminator3/1  "Reserved"
  Gain6/1 -> Terminator4/1  "Reserved"
  Gain3/1 -> Terminator1/1  "Reserved"
  Gain4/1 -> Terminator2/1  "Reserved"
  Gain2/1 -> Terminator/1  "Reserved"
  Gain1/1 -> WarningsActive/1  "WarningsActive"
  Gain/1 -> FaultActive/1  "FaultActive"
  Gain7/1 -> Terminator5/1  "Reserved"
  Gain8/1 -> SystemActive/1  "SystemActive"
  Gain9/1 -> SpTqLF/1  "SpTqLF"
  Gain10/1 -> SpTqRF/1  "SpTqRF"
  Gain11/1 -> SpTqLR/1  "SpTqLR"
  Gain12/1 -> SpTqRR/1  "SpTqRR"
  Gain14/1 -> Terminator7/1  "Reserved"
  Gain13/1 -> Terminator8/1  "Reserved"
  Gain15/1 -> Terminator6/1  "Reserved"
  SysStsBits/1 -> Extract Bits9/1, Extract Bits10/1, Extract Bits16/1, Extract Bits15/1, Extract Bits14/1, Extract Bits13/1, Extract Bits12/1, Extract Bits11/1, Extract Bits8/1, Extract Bits7/1, Extract Bits6/1, Extract Bits5/1, Extract Bits4/1, Extract Bits3/1, Extract Bits2/1, Extract Bits1/1
  Extract Bits16/1 -> Gain15/1
  Extract Bits14/1 -> Gain13/1
  Extract Bits15/1 -> Gain14/1
  Extract Bits13/1 -> Gain12/1
  Extract Bits12/1 -> Gain11/1
  Extract Bits11/1 -> Gain10/1
  Extract Bits9/1 -> Gain8/1
  Extract Bits10/1 -> Gain9/1
  Extract Bits2/1 -> Gain1/1
  Extract Bits5/1 -> Gain4/1
  Extract Bits1/1 -> Gain/1
  Extract Bits3/1 -> Gain2/1
  Extract Bits7/1 -> Gain6/1
  Extract Bits8/1 -> Gain7/1
  Extract Bits4/1 -> Gain3/1
  Extract Bits6/1 -> Gain5/1

== system CAVE_MachE_speedCtrl/Vehicle Under Test/Vehicle/Rototest and ORNL Interface/Get Wheel Spd Cmd Based on Wheel Dynamics/Whl Dynamics & Format CM Powertrain Signal/Diff Trq ==
  In1 : Inport
  Constant : Constant  Value=4.1
  Gain10 : Gain  Gain=0.5
  Product : Product  RndMeth=Zero
  Out1 : Outport
  wires:
  Gain10/1 -> Out1/1
  Constant/1 -> Product/1
  In1/1 -> Product/2
  Product/1 -> Gain10/1  "DiffTrq"

== system CAVE_MachE_speedCtrl/Vehicle Under Test/Vehicle/Rototest and ORNL Interface/Get Wheel Spd Cmd Based on Wheel Dynamics/Whl Dynamics & Format CM Powertrain Signal/Subsystem ==
  BrakeTorq : Inport
  <Car Trq_T2WFL> : Inport  Port=2
  AxlTorq : Inport  Port=3
  Fx : Inport  Port=4
  Add1 : Sum  Inputs=--+
  Add2 : Sum  Inputs=-+
  Constant : Constant  Value=0
  Constant9 : Constant  Value=0.3135
  MATLAB Function : MATLAB Function  TreatAsAtomicUnit=on
  Memory : Memory
  Output Damping : Gain  Gain=0  SaturateOnIntegerOverflow=on  OutDataTypeStr=Inherit: Same as input  ParamDataTypeStr=Inherit: Same as input
  Product3 : Product  Inputs=**
  Saturation : Saturate  UpperLimit=inf  LowerLimit=0  ZeroCross=off
  Sum : Sum  Inputs=--
  Sum3 : Sum  Inputs=-++
  Switch : Switch  Criteria=u2 > Threshold
  WheelInertia : Subsystem
  WheelInertia1 : Subsystem
  omega wheel : Integrator  ContinuousStateAttributes='omegaWheel'
  rotv FL : Outport
  wires:
  Sum3/1 -> WheelInertia/1(In1)
  BrakeTorq/1 -> Sum3/1
  MATLAB Function/1(switchFlag) -> Switch/2  "Flag1"
  Constant/1 -> Switch/1
  Memory/1 -> MATLAB Function/2(wheelSpd)
  Add2/1 -> Saturation/1
  [RhoZ1] -> Add2/1
  Constant9/1 -> Add2/2
  AxlTorq/1 -> Add1/1, MATLAB Function/1(axleTorq), Sum3/3
  <Car Trq_T2WFL>/1 -> Add1/2, Sum3/2
  Product3/1 -> Add1/3
  Saturation/1 -> Product3/2
  Add1/1 -> WheelInertia1/1(In1)
  Switch/1 -> omega wheel/1
  omega wheel/1 -> Memory/1, Output Damping/1, rotv FL/1
  Output Damping/1 -> Sum/2
  WheelInertia1/1(axleTorq) -> Sum/1  "rota"
  Sum/1 -> Switch/3
  [Fx1] -> Product3/1
